simulink model "Boat_model_paper"  (Simulink 6.6)
settings: Solver=ode3  StartTime=0.0  StopTime=10000  FixedStep=.01  RelTol=1e-3
values from neighbouring files (symbols this model uses):
  C_d_sea_surge = 340    [boat_constants.m]
  cg_x = .0508    (= 0.0508)    [boat_constants.m]
  cg_z = .0508    (= 0.0508)    [boat_constants.m]
  d_prop = .4572    (= 0.4572)    [boat_constants.m]
  e_0 = 0    [boat_constants.m]
  I_xx = mass/12*(3^2+4^2)    (= 1145.83333333)    [boat_constants.m]
  I_zz = mass/12*(13^2+3^2)    (= 8158.33333333)    [boat_constants.m]
  K_t = 0.5    [boat_constants.m]
  mass = 550    [boat_constants.m]
  n_0 = 0    [boat_constants.m]
  proportional_band = .5    (= 0.5)    [boat_constants.m]
  psi_0 = 0    [boat_constants.m]
  rho_w = 1.03e3    (= 1030)    [boat_constants.m]
  rudder_angle_dot_max = 10    [boat_constants.m]
  rudder_angle_max = 1    [boat_constants.m]
  wheelbase = 3.27    [boat_constants.m]
undefined symbols (not defined in the file or in its folder): render_boat
libraries: vrlib x1, simulink x1
settings Model: Creator=Administrator  LastModifiedBy=Administrator
settings DebuggingCC: AlgebraicLoopMsg=error

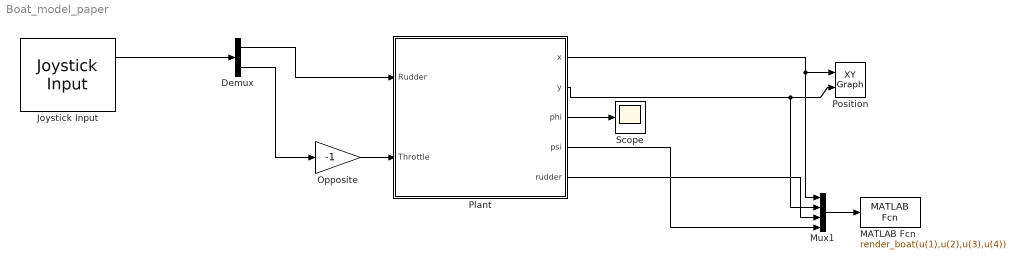
== system Boat_model_paper ==
  Demux : Demux  Outputs=3
  Joystick Input : vrlib/Joystick Input  joyid=1  adjustports=on  forcefeed=off
  MATLAB Fcn : MATLABFcn  MATLABFcn=render_boat(u(1),u(2),u(3),u(4))  OutputDimensions=0  Output1D=off
  Mux1 : Mux
  Opposite : Gain  Gain=-1
  Plant : Subsystem
  Position : simulink/Sinks/XY Graph  SystemSampleTime=-1  xmin=-1000  xmax=1000  ymin=-1000  ymax=1000  st=-1
  Scope : Scope
  wires:
  Demux/1 -> Plant/1(Rudder)
  Demux/3 -> Opposite/1
  Joystick Input/1 -> Demux/1
  Mux1/1 -> MATLAB Fcn/1
  Opposite/1 -> Plant/2(Throttle)
  Plant/1(x) -> Mux1/1, Position/1
  Plant/2(y) -> Position/2, Mux1/2
  Plant/4(psi) -> Mux1/4
  Plant/3(phi) -> Scope/1
  Plant/5(rudder) -> Mux1/3

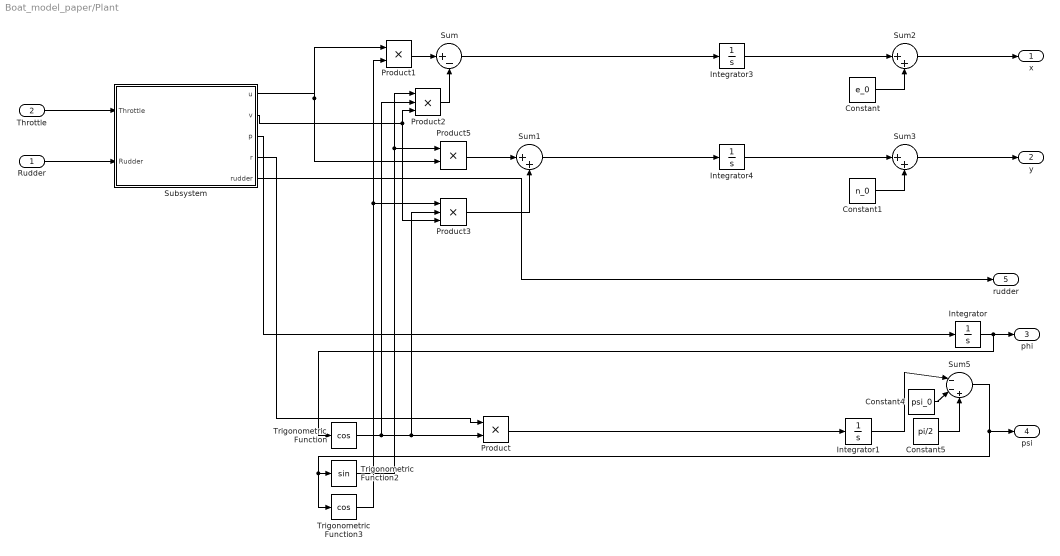
== system Boat_model_paper/Plant ==
  Rudder : Inport
  Throttle : Inport  Port=2
  Constant : Constant  Value=e_0
  Constant1 : Constant  Value=n_0
  Constant4 : Constant  Value=psi_0
  Constant5 : Constant  Value=pi/2
  Integrator{,1,3..4} (4 alike) : Integrator
  Product : Product  RndMeth=Zero
  Product1 : Product  RndMeth=Zero
  Product2 : Product  Inputs=3  RndMeth=Zero
  Product3 : Product  Inputs=3  RndMeth=Zero
  Product5 : Product  RndMeth=Zero
  Subsystem : Subsystem
  Sum : Sum  Inputs=|+-
  Sum1 : Sum  Inputs=|++
  Sum2 : Sum  Inputs=|++
  Sum3 : Sum  Inputs=|++
  Sum5 : Sum  Inputs=|--+
  Trigonometric Function : Trigonometry  Operator=cos
  Trigonometric Function2 : Trigonometry
  Trigonometric Function3 : Trigonometry  Operator=cos
  x : Outport
  y : Outport  Port=2
  phi : Outport  Port=3
  psi : Outport  Port=4
  rudder : Outport  Port=5
  wires:
  Throttle/1 -> Subsystem/1(Throttle)
  Rudder/1 -> Subsystem/2(Rudder)
  Subsystem/3(p) -> Integrator/1
  Trigonometric Function/1 -> Product/2, Product3/2, Product2/2
  Subsystem/4(r) -> Product/1
  Product/1 -> Integrator1/1
  Product2/1 -> Sum/2
  Product1/1 -> Sum/1
  Subsystem/1(u) -> Product1/1, Product5/2
  Trigonometric Function3/1 -> Product1/2, Product3/1
  Trigonometric Function2/1 -> Product2/1, Product5/1
  Subsystem/2(v) -> Product2/3, Product3/3
  Product5/1 -> Sum1/1
  Product3/1 -> Sum1/2
  Sum/1 -> Integrator3/1
  Integrator/1 -> phi/1, Trigonometric Function/1
  Constant4/1 -> Sum5/2
  Constant5/1 -> Sum5/3
  Integrator1/1 -> Sum5/1
  Sum5/1 -> psi/1, Trigonometric Function2/1, Trigonometric Function3/1
  Subsystem/5(rudder) -> rudder/1
  Constant/1 -> Sum2/2
  Integrator3/1 -> Sum2/1
  Sum2/1 -> x/1
  Integrator4/1 -> Sum3/1
  Constant1/1 -> Sum3/2
  Sum3/1 -> y/1
  Sum1/1 -> Integrator4/1

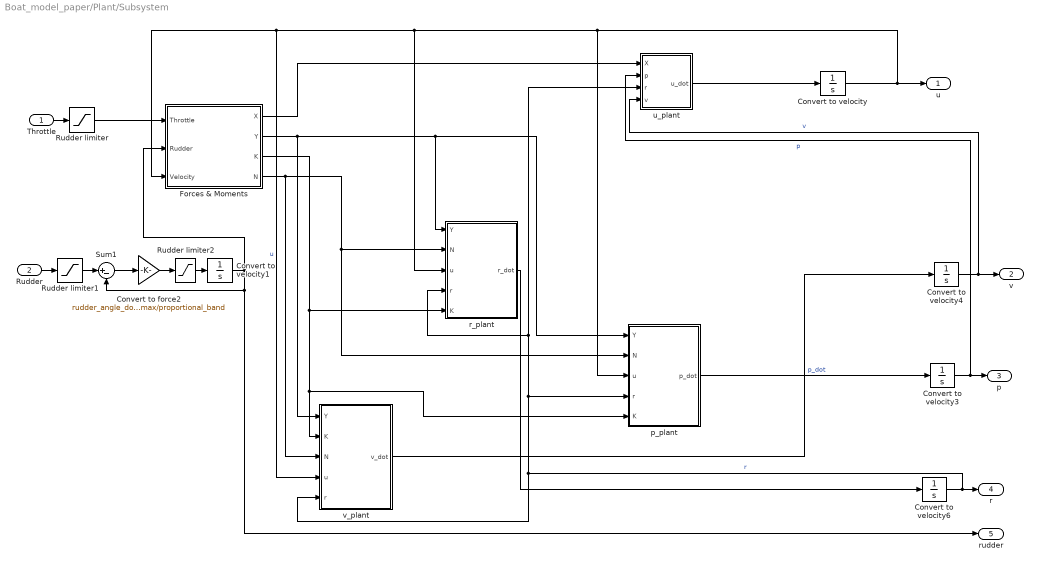
== system Boat_model_paper/Plant/Subsystem ==
  Throttle : Inport
  Rudder : Inport  Port=2
  Convert to force2 : Gain  Gain=rudder_angle_dot_max/proportional_band
  Convert to velocity{,3..4,6} (4 alike) : Integrator
  Convert to velocity1 : Integrator  LimitOutput=on  UpperSaturationLimit=rudder_angle_max  LowerSaturationLimit=-rudder_angle_max
  Forces & Moments : Subsystem
  Rudder limiter : Saturate  UpperLimit=1  LowerLimit=0
  Rudder limiter1 : Saturate  UpperLimit=rudder_angle_max  LowerLimit=-rudder_angle_max
  Rudder limiter2 : Saturate  UpperLimit=rudder_angle_dot_max  LowerLimit=-rudder_angle_dot_max
  Sum1 : Sum  Inputs=|+-
  p_plant : Subsystem
  r_plant : Subsystem
  u_plant : Subsystem
  v_plant : Subsystem
  u : Outport
  v : Outport  Port=2
  p : Outport  Port=3
  r : Outport  Port=4
  rudder : Outport  Port=5
  wires:
  Convert to velocity/1 -> u/1, r_plant/3(u), Forces & Moments/3(Velocity), v_plant/4(u), p_plant/3(u)  "u"
  Forces & Moments/1(X) -> u_plant/1(X)
  Rudder/1 -> Rudder limiter1/1
  Throttle/1 -> Rudder limiter/1
  Convert to velocity4/1 -> v/1, u_plant/4(v)  "v"
  p_plant/1(p_dot) -> Convert to velocity3/1  "p_dot"
  Convert to velocity3/1 -> p/1, u_plant/2(p)  "p"
  Convert to velocity6/1 -> r/1, v_plant/5(r), u_plant/3(r), r_plant/4(r), p_plant/4(r)  "r"
  u_plant/1(u_dot) -> Convert to velocity/1
  Forces & Moments/4(N) -> v_plant/3(N), r_plant/2(N), p_plant/2(N)
  Forces & Moments/3(K) -> v_plant/2(K), p_plant/5(K), r_plant/5(K)
  Forces & Moments/2(Y) -> v_plant/1(Y), r_plant/1(Y), p_plant/1(Y)
  v_plant/1(v_dot) -> Convert to velocity4/1
  r_plant/1(r_dot) -> Convert to velocity6/1
  Rudder limiter/1 -> Forces & Moments/1(Throttle)
  Convert to velocity1/1 -> Sum1/2, rudder/1, Forces & Moments/2(Rudder)
  Sum1/1 -> Convert to force2/1
  Rudder limiter1/1 -> Sum1/1
  Rudder limiter2/1 -> Convert to velocity1/1
  Convert to force2/1 -> Rudder limiter2/1

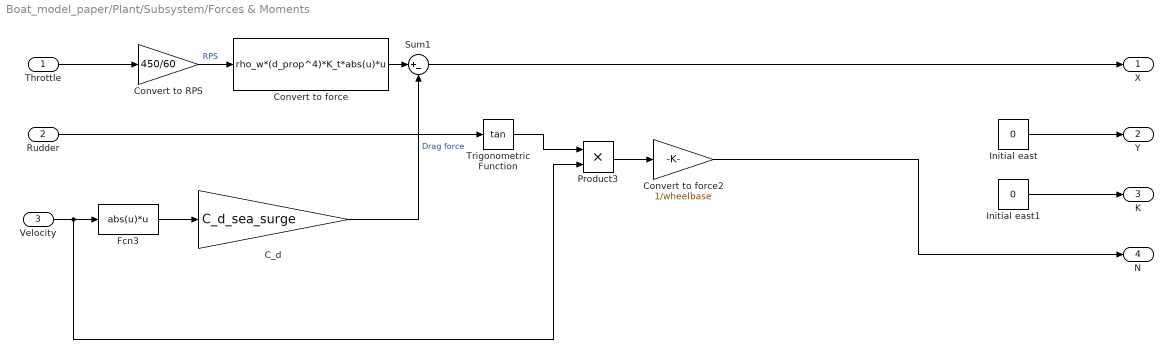
== system Boat_model_paper/Plant/Subsystem/Forces & Moments ==
  Throttle : Inport
  Rudder : Inport  Port=2
  Velocity : Inport  Port=3
  C_d : Gain  Gain=C_d_sea_surge
  Convert to RPS : Gain  Gain=450/60
  Convert to force2 : Gain  Gain=1/wheelbase
  Convert to force : Fcn  Expr=rho_w*(d_prop^4)*K_t*abs(u)*u
  Fcn3 : Fcn  Expr=abs(u)*u
  Initial east : Constant  Value=0
  Initial east1 : Constant  Value=0
  Product3 : Product  RndMeth=Zero
  Sum1 : Sum  Inputs=|+-
  Trigonometric Function : Trigonometry  Operator=tan  OutputSignalType=real
  X : Outport
  Y : Outport  Port=2
  K : Outport  Port=3
  N : Outport  Port=4
  wires:
  Convert to RPS/1 -> Convert to force/1  "RPS"
  Fcn3/1 -> C_d/1
  C_d/1 -> Sum1/2  "Drag force"
  Convert to force/1 -> Sum1/1
  Velocity/1 -> Fcn3/1, Product3/2
  Throttle/1 -> Convert to RPS/1
  Sum1/1 -> X/1
  Rudder/1 -> Trigonometric Function/1
  Product3/1 -> Convert to force2/1
  Trigonometric Function/1 -> Product3/1
  Convert to force2/1 -> N/1
  Initial east/1 -> Y/1
  Initial east1/1 -> K/1

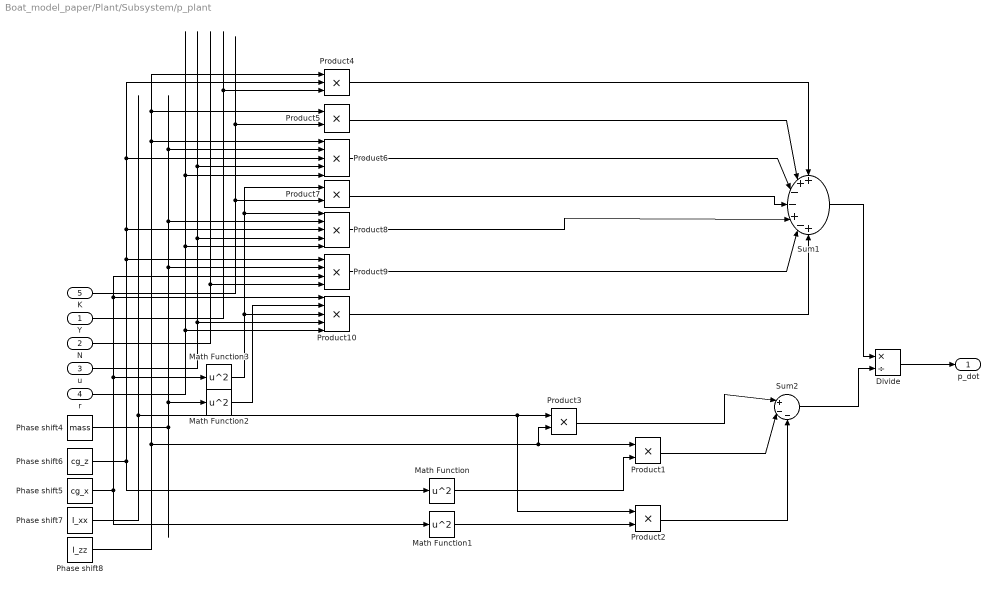
== system Boat_model_paper/Plant/Subsystem/p_plant ==
  Y : Inport
  N : Inport  Port=2
  u : Inport  Port=3
  r : Inport  Port=4
  K : Inport  Port=5
  Divide : Product  Inputs=*/  OutScaling=2^-10
  Math Function{,1..3} (4 alike) : Math  Operator=square  SaturateOnIntegerOverflow=on
  Phase shift4 : Constant  Value=mass
  Phase shift5 : Constant  Value=cg_x
  Phase shift6 : Constant  Value=cg_z
  Phase shift7 : Constant  Value=I_xx
  Phase shift8 : Constant  Value=I_zz
  Product{1..3,5,7} (5 alike) : Product  RndMeth=Zero
  Product10 : Product  Inputs=5  RndMeth=Zero
  Product4 : Product  Inputs=3  RndMeth=Zero
  Product6 : Product  Inputs=5  RndMeth=Zero
  Product8 : Product  Inputs=5  RndMeth=Zero
  Product9 : Product  Inputs=4  RndMeth=Zero
  Sum1 : Sum  Inputs=++--+-+
  Sum2 : Sum  Inputs=|+--
  p_dot : Outport
  wires:
  Sum1/1 -> Divide/1
  Divide/1 -> p_dot/1
  r/1 -> Product6/5, Product8/5, Product10/5
  u/1 -> Product6/4, Product8/4, Product10/4
  N/1 -> Product9/4
  Y/1 -> Product4/3
  Sum2/1 -> Divide/2
  Phase shift7/1 -> Product3/1, Product2/1
  Phase shift8/1 -> Product3/2, Product1/1, Product4/1, Product5/1, Product6/1
  Product3/1 -> Sum2/1
  Phase shift6/1 -> Math Function/1, Product4/2, Product6/3, Product8/3, Product9/1
  Math Function/1 -> Product1/2
  Product1/1 -> Sum2/2
  Math Function1/1 -> Product2/2
  Product2/1 -> Sum2/3
  Phase shift4/1 -> Product6/2, Product8/2, Product9/2, Math Function2/1
  K/1 -> Product5/2, Product7/2
  Phase shift5/1 -> Math Function1/1, Math Function3/1, Product9/3, Product10/1
  Product4/1 -> Sum1/1
  Product5/1 -> Sum1/2
  Product6/1 -> Sum1/3
  Product7/1 -> Sum1/4
  Math Function3/1 -> Product7/1, Product8/1, Product10/3
  Product8/1 -> Sum1/5
  Product9/1 -> Sum1/6
  Product10/1 -> Sum1/7
  Math Function2/1 -> Product10/2

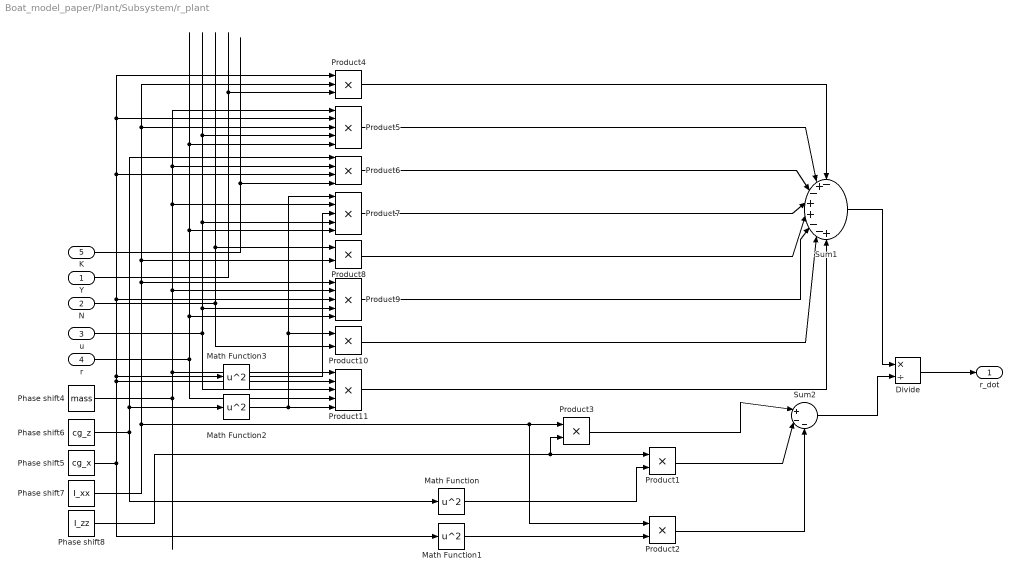
== system Boat_model_paper/Plant/Subsystem/r_plant ==
  Y : Inport
  N : Inport  Port=2
  u : Inport  Port=3
  r : Inport  Port=4
  K : Inport  Port=5
  Divide : Product  Inputs=*/  OutScaling=2^-10
  Math Function{,1..3} (4 alike) : Math  Operator=square  SaturateOnIntegerOverflow=on
  Phase shift4 : Constant  Value=mass
  Phase shift5 : Constant  Value=cg_x
  Phase shift6 : Constant  Value=cg_z
  Phase shift7 : Constant  Value=I_xx
  Phase shift8 : Constant  Value=I_zz
  Product{1..3,8,10} (5 alike) : Product  RndMeth=Zero
  Product{5,7,9,11} (4 alike) : Product  Inputs=5  RndMeth=Zero
  Product4 : Product  Inputs=3  RndMeth=Zero
  Product6 : Product  Inputs=4  RndMeth=Zero
  Sum1 : Sum  Inputs=-+-++--+
  Sum2 : Sum  Inputs=|+--
  r_dot : Outport
  wires:
  Sum1/1 -> Divide/1
  Divide/1 -> r_dot/1
  r/1 -> Product5/5, Product7/5, Product9/5, Product11/4
  u/1 -> Product5/4, Product7/4, Product9/4, Product11/3
  N/1 -> Product8/1, Product10/2
  Y/1 -> Product4/3
  Sum2/1 -> Divide/2
  Phase shift7/1 -> Product3/1, Product2/1, Product4/2, Product5/3, Product8/2, Product9/1
  Phase shift8/1 -> Product3/2, Product1/1
  Product3/1 -> Sum2/1
  Phase shift6/1 -> Math Function/1, Product6/1, Math Function2/1
  Math Function/1 -> Product1/2
  Product1/1 -> Sum2/2
  Math Function1/1 -> Product2/2
  Phase shift5/1 -> Math Function1/1, Product4/1, Product5/2, Product6/3, Product9/3, Math Function3/1, Product11/2
  Product2/1 -> Sum2/3
  Phase shift4/1 -> Product5/1, Product6/2, Product7/2, Product9/2, Product11/1
  Product4/1 -> Sum1/1
  Product5/1 -> Sum1/2
  Product6/1 -> Sum1/3
  K/1 -> Product6/4
  Product7/1 -> Sum1/4
  Math Function2/1 -> Product7/1, Product10/1, Product11/5
  Product8/1 -> Sum1/5
  Product9/1 -> Sum1/6
  Product10/1 -> Sum1/7
  Product11/1 -> Sum1/8
  Math Function3/1 -> Product7/3

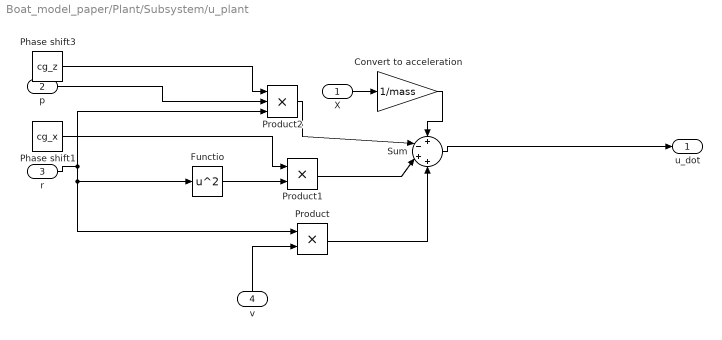
== system Boat_model_paper/Plant/Subsystem/u_plant ==
  X : Inport
  p : Inport  Port=2
  r : Inport  Port=3
  v : Inport  Orientation=up  Port=4
  Convert to acceleration : Gain  Gain=1/mass
  Functio : Math  Operator=square  SaturateOnIntegerOverflow=on
  Phase shift1 : Constant  Value=cg_x
  Phase shift3 : Constant  Value=cg_z
  Product : Product  RndMeth=Zero
  Product1 : Product  RndMeth=Zero
  Product2 : Product  Inputs=3  RndMeth=Zero
  Sum : Sum  Inputs=+-++
  u_dot : Outport
  wires:
  Product/1 -> Sum/4
  Functio/1 -> Product1/2
  Product1/1 -> Sum/3
  Product2/1 -> Sum/2
  Phase shift3/1 -> Product2/1
  p/1 -> Product2/2
  Phase shift1/1 -> Product1/1
  r/1 -> Product/1, Product2/3, Functio/1
  v/1 -> Product/2
  Sum/1 -> u_dot/1
  Convert to acceleration/1 -> Sum/1
  X/1 -> Convert to acceleration/1

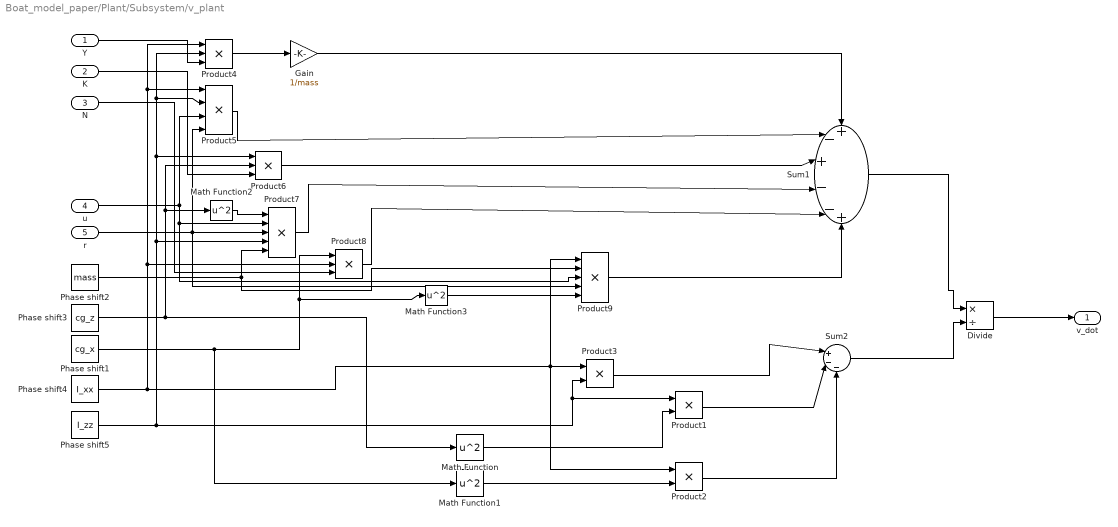
== system Boat_model_paper/Plant/Subsystem/v_plant ==
  Y : Inport
  K : Inport  Port=2
  N : Inport  Port=3
  u : Inport  Port=4
  r : Inport  Port=5
  Divide : Product  Inputs=*/  OutScaling=2^-10
  Gain : Gain  Gain=1/mass
  Math Function{,1..3} (4 alike) : Math  Operator=square  SaturateOnIntegerOverflow=on
  Phase shift1 : Constant  Value=cg_x
  Phase shift2 : Constant  Value=mass
  Phase shift3 : Constant  Value=cg_z
  Phase shift4 : Constant  Value=I_xx
  Phase shift5 : Constant  Value=I_zz
  Product1 : Product  RndMeth=Zero
  Product2 : Product  RndMeth=Zero
  Product3 : Product  RndMeth=Zero
  Product4 : Product  Inputs=3  RndMeth=Zero
  Product5 : Product  Inputs=4  RndMeth=Zero
  Product6 : Product  Inputs=3  RndMeth=Zero
  Product7 : Product  Inputs=5  RndMeth=Zero
  Product8 : Product  Inputs=3  RndMeth=Zero
  Product9 : Product  Inputs=5  RndMeth=Zero
  Sum1 : Sum  Inputs=+-+--+
  Sum2 : Sum  Inputs=|+--
  v_dot : Outport
  wires:
  Divide/1 -> v_dot/1
  Sum2/1 -> Divide/2
  Phase shift4/1 -> Product3/1, Product2/1, Product9/1, Product4/1, Product5/1, Product8/2
  Phase shift5/1 -> Product3/2, Product1/1, Product4/2, Product5/2, Product6/1, Product7/4
  Product3/1 -> Sum2/1
  Phase shift3/1 -> Math Function/1, Product6/2, Math Function2/1
  Math Function/1 -> Product1/2
  Product1/1 -> Sum2/2
  Math Function1/1 -> Product2/2
  Phase shift1/1 -> Math Function1/1, Product8/1, Math Function3/1
  Product2/1 -> Sum2/3
  Y/1 -> Product4/3
  Product4/1 -> Gain/1
  Gain/1 -> Sum1/1
  u/1 -> Product5/3, Product7/2, Product9/3
  r/1 -> Product5/4, Product7/3, Product9/4
  Product5/1 -> Sum1/2
  Product6/1 -> Sum1/3
  K/1 -> Product6/3
  Phase shift2/1 -> Product7/5, Product9/2
  Math Function2/1 -> Product7/1
  Product7/1 -> Sum1/4
  Product8/1 -> Sum1/5
  N/1 -> Product8/3
  Product9/1 -> Sum1/6
  Math Function3/1 -> Product9/5
  Sum1/1 -> Divide/1
